simulink model "CH4_3D3"  (R2021b)
settings: Solver=ode45  StartTime=0.0  StopTime=3  RelTol=1e-3  EnableMultiTasking=on
undefined symbols (not defined in the file or in its folder): j
settings Model: Creator=my2  LastModifiedBy=82102
settings SolverCC: AlgebraicLoopSolver=TrustRegion
settings DataIOCC: LimitDataPoints=on  SaveFormat=Array  SignalLoggingSaveFormat=ModelDataLogs  ReturnWorkspaceOutputs=off
settings OptimizationCC: ExpressionDepthLimit=2147483647  LifeSpan=inf
settings DebuggingCC: UnderspecifiedInitializationDetection=Classic  MergeDetectMultiDrivingBlocksExec=none  SolverPrmCheckMsg=warning  FcnCallInpInsideContextMsg=warning  SFUnexpectedBacktrackingDiag=warning  SFNoUnconditionalDefaultTransitionDiag=warning  SFExecutionAtInitializationDiag=none  SFMachineParentedDataDiag=warning  ArithmeticOperatorsInVariantConditions=warning
settings HardwareCC: ProdBitPerPointer=32  ProdBitPerSizeT=32  ProdBitPerPtrDiffT=32  ProdLargestAtomicFloat=None  ProdIntDivRoundTo=Undefined  ProdEndianess=Unspecified  ProdWordSize=32  ProdHWDeviceType=32-bit Generic
settings ModelReferenceCC: PropagateSignalLabelsOutOfModel=off
settings SFSimCC: SimUseLocalCustomCode=off  CustomCodeUndefinedFunction=UseInterfaceOnly
settings RTWCC: RTWUseLocalCustomCode=off
settings CodeAppCC: StateflowObjectComments=on
settings GRTTargetCC: TargetLangStandard=C89/C90 (ANSI)  CombineOutputUpdateFcns=off  GRTInterface=on
settings ConfigComp: CovMetricSettings=dw  CovSaveCumulativeToWorkspaceVar=on  CovSaveSingleToWorkspaceVar=on  CovExternalEMLEnable=off

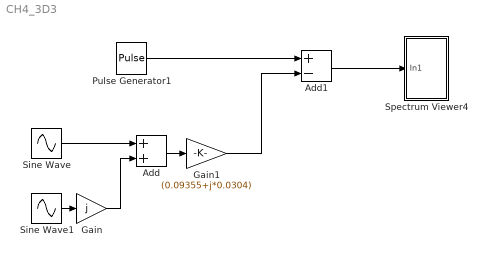
== system CH4_3D3 ==
  Add : Sum
  Add1 : Sum  Inputs=+-
  Gain : Gain  Gain=j
  Gain1 : Gain  Gain=(0.09355+j*0.0304)
  Pulse Generator1 : DiscretePulseGenerator  PulseType=Time based  Period=5e-4  PulseWidth=10
  Sine Wave : Sin  Frequency=(2*pi/5e-4)  Phase=pi/2  SampleTime=0
  Sine Wave1 : Sin  Amplitude=-1  Frequency=(2*pi/5e-4)  SampleTime=0
  Spectrum Viewer4 : Subsystem
  wires:
  Sine Wave1/1 -> Gain/1
  Sine Wave/1 -> Add/1
  Gain/1 -> Add/2
  Add/1 -> Gain1/1
  Pulse Generator1/1 -> Add1/1
  Gain1/1 -> Add1/2
  Add1/1 -> Spectrum Viewer4/1(In1)

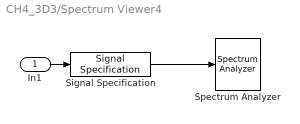
== system CH4_3D3/Spectrum Viewer4 ==
  In1 : Inport
  Signal Specification : SignalSpecification  SampleTime=1/16e4
  Spectrum Analyzer : SpectrumAnalyzer
  wires:
  In1/1 -> Signal Specification/1
  Signal Specification/1 -> Spectrum Analyzer/1
